simulink model "T3"  (R2024a)
settings: Solver=VariableStepAuto  StartTime=0.0  StopTime=10.0  RelTol=1e-3
libraries: cstblocks x1
settings Model: NumberOfSteps=2  Creator=PMYLS  LastModifiedBy=PMYLS

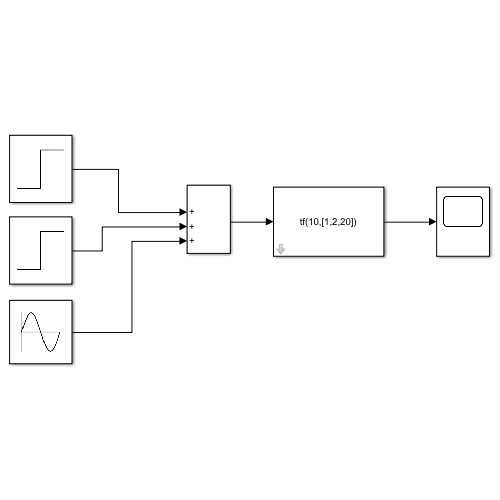
[thumbnail: Simulink's stored preview of the top-level diagram]
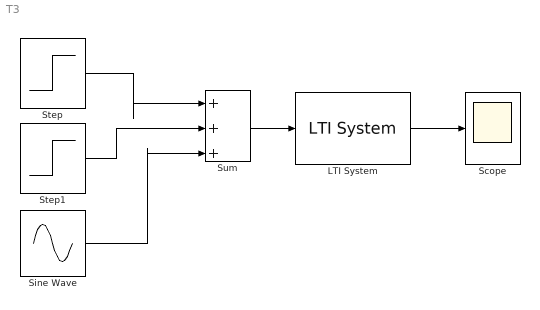
== system T3 ==
  LTI System : cstblocks/LTI System  sys=tf(10,[1,2,20])  IC=[]  PadeOrder=0
  Scope : Scope
  Sine Wave : Sin  Frequency=2*pi  SampleTime=0
  Step : Step  Time=0  SampleTime=0
  Step1 : Step  Time=5  After=2  SampleTime=0
  Sum : Sum  Inputs=|+++
  wires:
  LTI System/1 -> Scope/1
  Step1/1 -> Sum/2
  Step/1 -> Sum/1
  Sine Wave/1 -> Sum/3
  Sum/1 -> LTI System/1
